simulink model "Const_VF_Openloop"  (R2023a)
settings: Solver=VariableStepAuto  StartTime=0.0  StopTime=10.0  MaxStep=.00001  RelTol=1e-3
values from neighbouring files (symbols this model uses):
  B = .005752    (= 0.005752)    [Parameters.m]
  J = .02    (= 0.02)    [Parameters.m]
  offset = Vph_p-(slope*Freq)    [Parameters.m]
  P = 4    [Parameters.m]
  slope = (Vph_p-VF_boost)/(Freq-1)    [Parameters.m]
  Te_rated = Prated/Wr_rated    (= 20.3536435794)    [Parameters.m]
  Vph_p = VLL_p/sqrt(3)    [Parameters.m]
  Wslip_rated = Ws_rated-Wr_rated    (= 5.23598775598)    [Parameters.m]
libraries: spsMosfetLib x12, spsAsynchronousMachineSIUnitsLib x2, spsDCVoltageSourceLib x2, slpidlib x2, spsTriangleGeneratorLib x2, SignalEditorBlockLib x1, sps_lib x1
settings Model: Creator=User  LastModifiedBy=User
settings SolverCC: ConsecutiveZCsStepRelTol=1000*128*eps  MaxConsecutiveZCs=2000
settings DebuggingCC: IgnoredZcDiagnostic=none

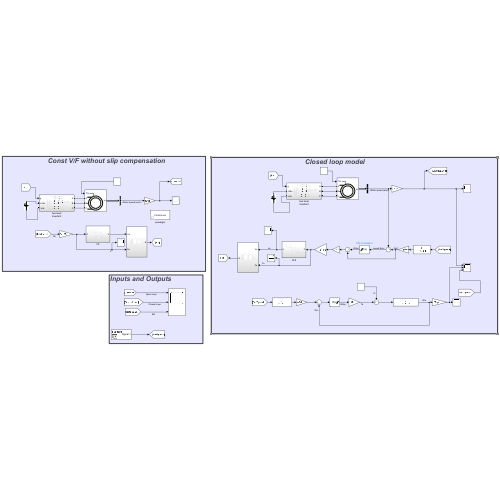
[thumbnail: Simulink's stored preview of the top-level diagram]
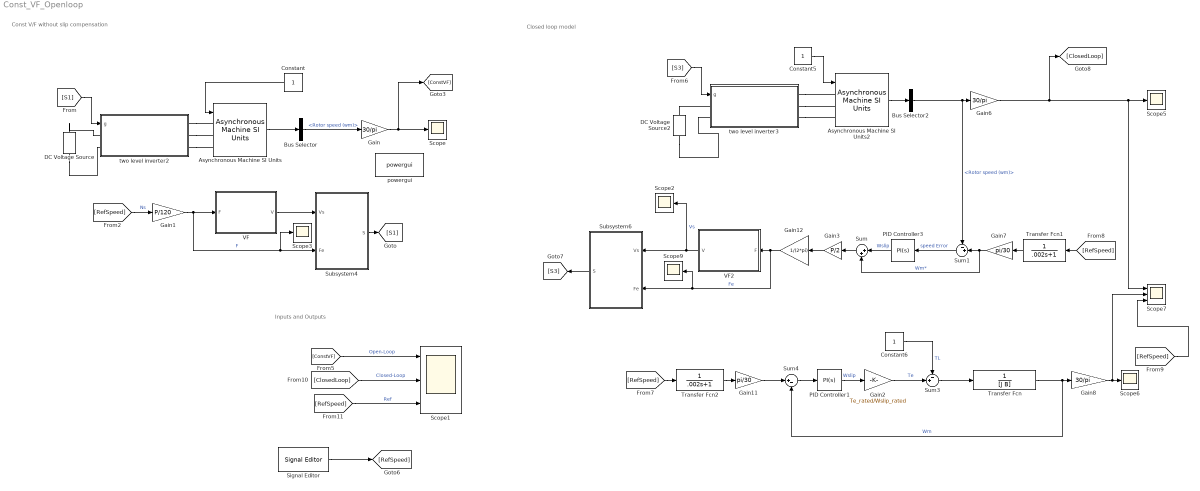
== system Const_VF_Openloop ==
  note: Inputs and Outputs
  note: Const V/F without slip compensation
  note: Closed loop model
  Asynchronous Machine SI Units : spsAsynchronousMachineSIUnitsLib/Asynchronous Machine SI Units  RotorType=Squirrel-cage  PresetModel="01:  5 HP   460 V 60Hz 1750 RPM"  MechanicalLoad=Torque Tm  ShowDetailedParameters=on  ReferenceFrame=Stationary  Units=SI  MeasurementBus=off  NominalParameters=[3730 460 60]  VoltageRatio=1  Stator=[1.115 0.005974]  Rotor=[1.083 0.005974]  Cage1=[0.4155 0.002066]  Cage2=[0.4168 0.0003495]  Lm=0.2037  Mechanical=[0.02 0.005752 2]  PolePairs=2  InitialConditions=[1 0 0 0 0 0 0 0]  SimulateSaturation=off  Saturation=[14.03593122, 27.81365428, 53.79336849, 72.68890987, 97.98006896, 148.6815601, 215.7428561, 302.9841135, 428.7778367 ; 230, 322, 414, 460, 506, 552, 598, 644, 690]  LoadFlowParameters=1492000  TsPowergui=0  TsBlock=-1  IterativeModel=Trapezoidal non iterative  IterativeDiscreteModel=Trapezoidal non iterative  Pmec=1.492e+006
  Asynchronous Machine SI Units2 : spsAsynchronousMachineSIUnitsLib/Asynchronous Machine SI Units  RotorType=Squirrel-cage  PresetModel="01:  5 HP   460 V 60Hz 1750 RPM"  MechanicalLoad=Torque Tm  ShowDetailedParameters=on  ReferenceFrame=Stationary  Units=SI  MeasurementBus=off  NominalParameters=[3730 460 60]  VoltageRatio=1  Stator=[1.115 0.005974]  Rotor=[1.083 0.005974]  Cage1=[0.4155 0.002066]  Cage2=[0.4168 0.0003495]  Lm=0.2037  Mechanical=[0.02 0.005752 2]  PolePairs=2  InitialConditions=[1 0 0 0 0 0 0 0]  SimulateSaturation=off  Saturation=[14.03593122, 27.81365428, 53.79336849, 72.68890987, 97.98006896, 148.6815601, 215.7428561, 302.9841135, 428.7778367 ; 230, 322, 414, 460, 506, 552, 598, 644, 690]  LoadFlowParameters=1492000  TsPowergui=0  TsBlock=-1  IterativeModel=Trapezoidal non iterative  IterativeDiscreteModel=Trapezoidal non iterative  Pmec=1.492e+006
  Bus Selector : BusSelector  OutputSignals=Mechanical.Rotor speed (wm)
  Bus Selector2 : BusSelector  OutputSignals=Mechanical.Rotor speed (wm)
  Constant : Constant
  Constant5 : Constant
  Constant6 : Constant
  DC Voltage Source : spsDCVoltageSourceLib/DC Voltage Source  Amplitude=Vph_p  Measurements=None
  DC Voltage Source2 : spsDCVoltageSourceLib/DC Voltage Source  Amplitude=Vph_p  Measurements=None
  Gain : Gain  Gain=30/pi
  Gain1 : Gain  Gain=P/120
  Gain11 : Gain  Gain=pi/30
  Gain12 : Gain  Gain=1/(2*pi)
  Gain2 : Gain  Gain=Te_rated/Wslip_rated
  Gain3 : Gain  Gain=P/2
  Gain6 : Gain  Gain=30/pi
  Gain7 : Gain  Gain=pi/30
  Gain8 : Gain  Gain=30/pi
  PID Controller1 : slpidlib/PID Controller  Controller=PI  Form=Parallel  TimeDomain=Continuous-time  UseExternalTs=off  SampleTime=-1  IntegratorMethod=Forward Euler  FilterMethod=Forward Euler  ControllerParametersSource=internal  P=2.61459800352204  I=169.186564549332  UseKiTs=off  D=0  N=100  UseFilter=on  TunerSelectOption=Transfer Function Based (PID Tuner App)  InitialConditionSource=internal  InitialConditionForIntegrator=0  InitialConditionForFilter=0  DifferentiatorICPrevScaledInput=0  ExternalReset=none  TrackingMode=off  Kt=1  LimitOutput=on  SatLimitsSource=internal  UpperSaturationLimit=Wslip_rated  LowerSaturationLimit=0  LinearizeAsGain=on  AntiWindupMode=clamping  Kb=1  LimitIntegrator=off  UpperIntegratorSaturationLimit=inf  LowerIntegratorSaturationLimit=-inf  POutMin=[]  POutMax=[]  IOutMin=[]  IOutMax=[]  DOutMin=[]  DOutMax=[]  NOutMin=[]  NOutMax=[]  SumOutMin=[]  SumOutMax=[]  SaturationOutMin=[]  SaturationOutMax=[]  PParamMin=[]  PParamMax=[]  IParamMin=[]  IParamMax=[]  DParamMin=[]  DParamMax=[]  NParamMin=[]  NParamMax=[]  KbParamMin=[]  KbParamMax=[]  KtParamMin=[]  KtParamMax=[]  KbOutMin=[]  KbOutMax=[]  KtOutMin=[]  KtOutMax=[]  IntegratorOutMin=[]  IntegratorOutMax=[]  FilterOutMin=[]  FilterOutMax=[]  SumI1OutMin=[]  SumI1OutMax=[]  SumI2OutMin=[]  SumI2OutMax=[]  SumI3OutMin=[]  SumI3OutMax=[]  SumI4OutMin=[]  SumI4OutMax=[]  SumDOutMin=[]  SumDOutMax=[]  DifferentiatorOutMin=[]  DifferentiatorOutMax=[]  FilterDiffOutCoefMin=[]  FilterDiffOutCoefMax=[]  ReciprocalOutMin=[]  ReciprocalOutMax=[]  SumDenOutMin=[]  SumDenOutMax=[]  SumNumOutMin=[]  SumNumOutMax=[]  DivideOutMin=[]  DivideOutMax=[]  UdiffTsProdOutMin=[]  UdiffTsProdOutMax=[]  NTsProdOutMin=[]  NTsProdOutMax=[]  UintegralTsProdOutMin=[]  UintegralTsProdOutMax=[]  UngainTsProdOutMin=[]  UngainTsProdOutMax=[]  ClampingZeroOutDataTypeStr=Inherit: Inherit via back propagation  ClampingZeroOutMin=[]  ClampingZeroOutMax=[]  FilterDenConstantOutDataTypeStr=Inherit: Inherit via back propagation  FilterDenConstantOutMin=[]  FilterDenConstantOutMax=[]  PCopyOutDataTypeStr=Inherit: Inherit via back propagation  PCopyOutMin=[]  PCopyOutMax=[]  NCopyOutDataTypeStr=Inherit: Inherit via back propagation  NCopyOutMin=[]  NCopyOutMax=[]  IntegratorContinuousStateAttributes=''  IntegratorStateMustResolveToSignalObject=off  IntegratorRTWStateStorageClass=Auto  FilterContinuousStateAttributes=''  FilterStateMustResolveToSignalObject=off  FilterRTWStateStorageClass=Auto  ParallelPVariant=InternalParameters  IdealPVariant=Disabled  IVariant=InternalParameters  DVariant=Disabled  IntegratorVariant=Continuous  SatVariant=Enabled  AWVariant=ContClampingParallel  PCopyVariant=Disabled  TRVariant=Disabled  FdbkBlocksVariant=Forward  IdealPFdbkVariant=Disabled  SatFdbkVariant=Disabled  DerivativeFilterVariant=Disabled  NVariant=Disabled  NCopyVariant=Disabled_SignalSpec  FilterICVariant=Disabled  IntegratorICVariant=InternalICs  ExternalResetVariant=Disabled  TRSumVariant=Passthrough  SumFdbkVariant=Disabled  SumVariant=Sum_PI  TsampFilterVariant=InternalTs  TsampNgainVariant=Passthrough  TsampIntegralVariant=Disabled_SignalSpec  ExternalSaturationOutDataTypeStr=Inherit: Same as second input
  PID Controller3 : slpidlib/PID Controller  Controller=PI  Form=Parallel  TimeDomain=Continuous-time  UseExternalTs=off  SampleTime=-1  IntegratorMethod=Forward Euler  FilterMethod=Forward Euler  ControllerParametersSource=internal  P=2.61459800352204  I=169.186564549332  UseKiTs=off  D=0  N=100  UseFilter=on  TunerSelectOption=Transfer Function Based (PID Tuner App)  InitialConditionSource=internal  InitialConditionForIntegrator=0  InitialConditionForFilter=0  DifferentiatorICPrevScaledInput=0  ExternalReset=none  TrackingMode=off  Kt=1  LimitOutput=on  SatLimitsSource=internal  UpperSaturationLimit=Wslip_rated  LowerSaturationLimit=0  LinearizeAsGain=on  AntiWindupMode=clamping  Kb=1  LimitIntegrator=off  UpperIntegratorSaturationLimit=inf  LowerIntegratorSaturationLimit=-inf  POutMin=[]  POutMax=[]  IOutMin=[]  IOutMax=[]  DOutMin=[]  DOutMax=[]  NOutMin=[]  NOutMax=[]  SumOutMin=[]  SumOutMax=[]  SaturationOutMin=[]  SaturationOutMax=[]  PParamMin=[]  PParamMax=[]  IParamMin=[]  IParamMax=[]  DParamMin=[]  DParamMax=[]  NParamMin=[]  NParamMax=[]  KbParamMin=[]  KbParamMax=[]  KtParamMin=[]  KtParamMax=[]  KbOutMin=[]  KbOutMax=[]  KtOutMin=[]  KtOutMax=[]  IntegratorOutMin=[]  IntegratorOutMax=[]  FilterOutMin=[]  FilterOutMax=[]  SumI1OutMin=[]  SumI1OutMax=[]  SumI2OutMin=[]  SumI2OutMax=[]  SumI3OutMin=[]  SumI3OutMax=[]  SumI4OutMin=[]  SumI4OutMax=[]  SumDOutMin=[]  SumDOutMax=[]  DifferentiatorOutMin=[]  DifferentiatorOutMax=[]  FilterDiffOutCoefMin=[]  FilterDiffOutCoefMax=[]  ReciprocalOutMin=[]  ReciprocalOutMax=[]  SumDenOutMin=[]  SumDenOutMax=[]  SumNumOutMin=[]  SumNumOutMax=[]  DivideOutMin=[]  DivideOutMax=[]  UdiffTsProdOutMin=[]  UdiffTsProdOutMax=[]  NTsProdOutMin=[]  NTsProdOutMax=[]  UintegralTsProdOutMin=[]  UintegralTsProdOutMax=[]  UngainTsProdOutMin=[]  UngainTsProdOutMax=[]  ClampingZeroOutDataTypeStr=Inherit: Inherit via back propagation  ClampingZeroOutMin=[]  ClampingZeroOutMax=[]  FilterDenConstantOutDataTypeStr=Inherit: Inherit via back propagation  FilterDenConstantOutMin=[]  FilterDenConstantOutMax=[]  PCopyOutDataTypeStr=Inherit: Inherit via back propagation  PCopyOutMin=[]  PCopyOutMax=[]  NCopyOutDataTypeStr=Inherit: Inherit via back propagation  NCopyOutMin=[]  NCopyOutMax=[]  IntegratorContinuousStateAttributes=''  IntegratorStateMustResolveToSignalObject=off  IntegratorRTWStateStorageClass=Auto  FilterContinuousStateAttributes=''  FilterStateMustResolveToSignalObject=off  FilterRTWStateStorageClass=Auto  ParallelPVariant=InternalParameters  IdealPVariant=Disabled  IVariant=InternalParameters  DVariant=Disabled  IntegratorVariant=Continuous  SatVariant=Enabled  AWVariant=ContClampingParallel  PCopyVariant=Disabled  TRVariant=Disabled  FdbkBlocksVariant=Forward  IdealPFdbkVariant=Disabled  SatFdbkVariant=Disabled  DerivativeFilterVariant=Disabled  NVariant=Disabled  NCopyVariant=Disabled_SignalSpec  FilterICVariant=Disabled  IntegratorICVariant=InternalICs  ExternalResetVariant=Disabled  TRSumVariant=Passthrough  SumFdbkVariant=Disabled  SumVariant=Sum_PI  TsampFilterVariant=InternalTs  TsampNgainVariant=Passthrough  TsampIntegralVariant=Disabled_SignalSpec  ExternalSaturationOutDataTypeStr=Inherit: Same as second input
  Scope{,2..3,5..6,9} (6 alike) : Scope
  Scope1 : Scope  NumInputPorts=3
  Scope7 : Scope  NumInputPorts=3
  Signal Editor : SignalEditorBlockLib/Signal Editor  FileName=speedRef.mat  ActiveScenario=Scenario  ActiveSignal=Signal 1  IsBus=off  OutputBusObjectStr=Bus: BusObject  SampleTime=0  Interpolate=off  ZeroCross=off  OutputAfterFinalValue=Setting to zero  Unit=inherit  PreserveSignalName=on  ApplySigPropsToAllScenarios=on
  Subsystem4 : Subsystem
  Subsystem6 : Subsystem
  Sum : Sum  Inputs=|++
  Sum1 : Sum  Inputs=-+|
  Sum3 : Sum  Inputs=-+|
  Sum4 : Sum  Inputs=|+-
  Transfer Fcn : TransferFcn  Denominator=[J B]
  Transfer Fcn1 : TransferFcn  Denominator=[.002 1]
  Transfer Fcn2 : TransferFcn  Denominator=[.002 1]
  VF : Subsystem
  VF2 : Subsystem
  powergui : sps_lib/powergui  Priority=1  SimulationMode=Continuous  SampleTime=50e-6  frequency=60  Iterations=50  frequencyindice=60  Pbase=100e6  ErrMax=1e-4  UnitsV=kV  UnitsW=MW  buscounter=0  FunctionMessages=off  echomessages=off  EnableUseOfTLC=off  CurrentSourceSwitches=off  DisableSnubberDevices=off  DisableRonSwitches=off  DisableVfSwitches=off  DisplayEquations=off  AutomaticDiscreteSolvers=off  SolverType=Tustin/Backward Euler (TBE)  Interpol=off  ExternalGateDelay=off  methode=off  Ts=100  x0status=blocks  SPID=on  SwTol=0  HookPort=off  NonlinearTolerance=1e-4  nMaxIteration=100  ContinueOnMaxIteration=off  RestoreLinks=warning  ResistiveCurrentMeasurement=off  Frange=[0:2:500]  Ylog=off  Xlog=on  ShowGrid=off  save=off  variable=ZData  structure=0  ZoomFFT=off  StartTime=0.0  cycles=1  DisplayStyle=1  fundamental=60  FreqAxis=off  MaxFrequency=1000  frequencyindicesteady=1  RmsSteady=1  display=off
  two level inverter2 : Subsystem
  two level inverter3 : Subsystem
  wires:
  Asynchronous Machine SI Units/1 -> Bus Selector/1
  Bus Selector/1 -> Gain/1  "<Rotor speed (wm)>"
  Gain/1 -> [ConstVF], Scope/1
  [RefSpeed] -> Gain1/1  "Ns"
  Gain1/1 -> Scope3/1, Subsystem4/2(Fe), VF/1(F)  "F"
  VF/1(V) -> Subsystem4/1(Vs)
  Constant/1 -> Asynchronous Machine SI Units/1
  Subsystem4/1(S) -> [S1]
  [S1] -> two level inverter2/1(g)
  [S3] -> two level inverter3/1(g)
  Constant5/1 -> Asynchronous Machine SI Units2/1
  Gain6/1 -> [ClosedLoop], Scope7/1, Scope5/1
  Bus Selector2/1 -> Sum1/1, Gain6/1  "<Rotor speed (wm)>"
  Asynchronous Machine SI Units2/1 -> Bus Selector2/1
  Signal Editor/1 -> [RefSpeed]
  Gain7/1 -> Sum/2, Sum1/2  "Wm*"
  Gain12/1 -> VF2/1(F), Subsystem6/2(Fe), Scope9/1  "Fe"
  Sum3/1 -> Transfer Fcn/1
  Constant6/1 -> Sum3/1  "TL"
  Transfer Fcn/1 -> Sum4/2, Gain8/1  "Wm"
  Sum4/1 -> PID Controller1/1
  PID Controller1/1 -> Gain2/1  "Wslip"
  Gain8/1 -> Scope7/2, Scope6/1
  Gain11/1 -> Sum4/1
  [RefSpeed] -> Transfer Fcn2/1
  [RefSpeed] -> Scope7/3
  VF2/1(V) -> Scope2/1, Subsystem6/1(Vs)  "Vs"
  Subsystem6/1(S) -> [S3]
  [ConstVF] -> Scope1/1  "Open-Loop"
  [ClosedLoop] -> Scope1/2  "Closed-Loop"
  [RefSpeed] -> Scope1/3  "Ref"
  [RefSpeed] -> Transfer Fcn1/1
  Gain2/1 -> Sum3/2  "Te"
  Sum1/1 -> PID Controller3/1  "speed Error"
  PID Controller3/1 -> Sum/1  "Wslip"
  Sum/1 -> Gain3/1
  Transfer Fcn1/1 -> Gain7/1
  Transfer Fcn2/1 -> Gain11/1
  Gain3/1 -> Gain12/1
  connections:
  two level inverter2/RConn1 -- Asynchronous Machine SI Units/LConn1
  two level inverter2/RConn2 -- Asynchronous Machine SI Units/LConn2
  DC Voltage Source/RConn1 -- two level inverter2/LConn1
  DC Voltage Source/LConn1 -- two level inverter2/LConn2
  two level inverter2/RConn3 -- Asynchronous Machine SI Units/LConn3
  two level inverter3/RConn3 -- Asynchronous Machine SI Units2/LConn3
  DC Voltage Source2/RConn1 -- two level inverter3/LConn1
  two level inverter3/RConn1 -- Asynchronous Machine SI Units2/LConn1
  two level inverter3/RConn2 -- Asynchronous Machine SI Units2/LConn2
  DC Voltage Source2/LConn1 -- two level inverter3/LConn2

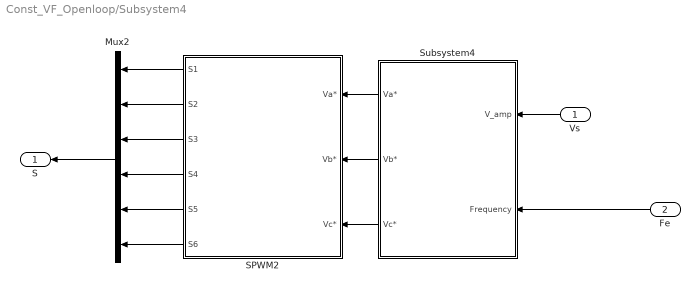
== system Const_VF_Openloop/Subsystem4 ==
  Vs : Inport
  Fe : Inport  Port=2
  Mux2 : Mux  Inputs=6
  SPWM2 : Subsystem
  Subsystem4 : Subsystem
  S : Outport
  wires:
  Mux2/1 -> S/1
  Fe/1 -> Subsystem4/2(Frequency)
  Vs/1 -> Subsystem4/1(V_amp)
  SPWM2/5(S5) -> Mux2/5
  Subsystem4/2(Vb*) -> SPWM2/2(Vb*)
  Subsystem4/1(Va*) -> SPWM2/1(Va*)
  SPWM2/6(S6) -> Mux2/6
  SPWM2/4(S4) -> Mux2/4
  SPWM2/1(S1) -> Mux2/1
  SPWM2/2(S2) -> Mux2/2
  SPWM2/3(S3) -> Mux2/3
  Subsystem4/3(Vc*) -> SPWM2/3(Vc*)

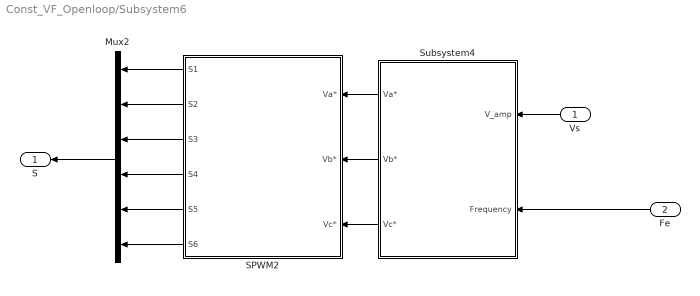
== system Const_VF_Openloop/Subsystem6 ==
  Vs : Inport
  Fe : Inport  Port=2
  Mux2 : Mux  Inputs=6
  SPWM2 : Subsystem
  Subsystem4 : Subsystem
  S : Outport
  wires:
  Subsystem4/3(Vc*) -> SPWM2/3(Vc*)
  SPWM2/3(S3) -> Mux2/3
  SPWM2/2(S2) -> Mux2/2
  SPWM2/1(S1) -> Mux2/1
  SPWM2/4(S4) -> Mux2/4
  SPWM2/6(S6) -> Mux2/6
  Subsystem4/1(Va*) -> SPWM2/1(Va*)
  Subsystem4/2(Vb*) -> SPWM2/2(Vb*)
  SPWM2/5(S5) -> Mux2/5
  Vs/1 -> Subsystem4/1(V_amp)
  Fe/1 -> Subsystem4/2(Frequency)
  Mux2/1 -> S/1

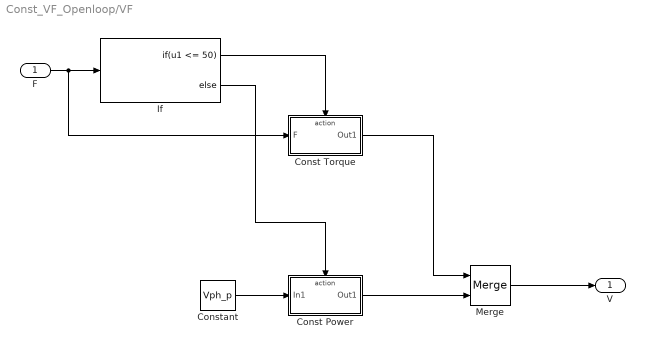
== system Const_VF_Openloop/VF ==
  F : Inport
  Const Power : Subsystem  TreatAsAtomicUnit=on
  Const Torque : Subsystem  TreatAsAtomicUnit=on
  Constant : Constant  Value=Vph_p
  If : If  IfExpression=u1 <= 50
  Merge : Merge
  V : Outport
  wires:
  F/1 -> Const Torque/1(F), If/1
  If/2 -> Const Power/Action
  Const Torque/1(Out1) -> Merge/1
  If/1 -> Const Torque/Action
  Merge/1 -> V/1
  Constant/1 -> Const Power/1(In1)
  Const Power/1(Out1) -> Merge/2

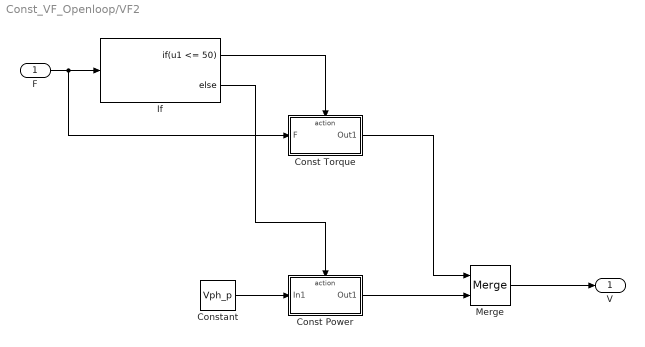
== system Const_VF_Openloop/VF2 ==
  F : Inport
  Const Power : Subsystem  TreatAsAtomicUnit=on
  Const Torque : Subsystem  TreatAsAtomicUnit=on
  Constant : Constant  Value=Vph_p
  If : If  IfExpression=u1 <= 50
  Merge : Merge
  V : Outport
  wires:
  Const Power/1(Out1) -> Merge/2
  Constant/1 -> Const Power/1(In1)
  Merge/1 -> V/1
  If/1 -> Const Torque/Action
  Const Torque/1(Out1) -> Merge/1
  If/2 -> Const Power/Action
  F/1 -> If/1, Const Torque/1(F)

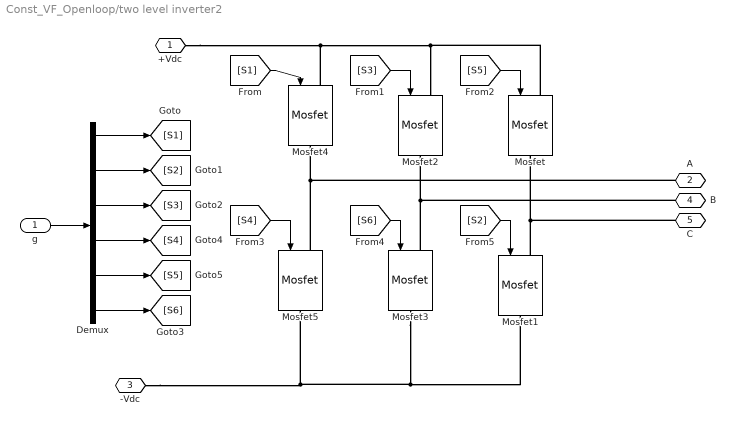
== system Const_VF_Openloop/two level inverter2 ==
  g : Inport
  Demux : Demux  Outputs=6
  Mosfet{,1..5} (6 alike) : spsMosfetLib/Mosfet  Ron=0.1  Lon=0  Rd=0.01  Vfd=0  IC=0  Rs=1e5  Cs=inf  Measurements=off
  +Vdc : PMIOPort  Side=Left
  A : PMIOPort  Port=2  Side=Right
  -Vdc : PMIOPort  Port=3  Side=Left
  B : PMIOPort  Port=4  Side=Right
  C : PMIOPort  Port=5  Side=Right
  wires:
  g/1 -> Demux/1
  Demux/1 -> [S1]
  Demux/2 -> [S2]
  Demux/3 -> [S3]
  Demux/4 -> [S4]
  Demux/5 -> [S5]
  Demux/6 -> [S6]
  [S1] -> Mosfet4/1
  [S3] -> Mosfet2/1
  [S5] -> Mosfet/1
  [S4] -> Mosfet5/1
  [S6] -> Mosfet3/1
  [S2] -> Mosfet1/1
  connections:
  Mosfet4/LConn1 -- +Vdc/RConn1 -- Mosfet/LConn1 -- Mosfet2/LConn1
  Mosfet3/RConn1 -- Mosfet1/RConn1 -- -Vdc/RConn1 -- Mosfet5/RConn1
  Mosfet1/LConn1 -- Mosfet/RConn1 -- C/RConn1
  Mosfet3/LConn1 -- B/RConn1 -- Mosfet2/RConn1
  A/RConn1 -- Mosfet5/LConn1 -- Mosfet4/RConn1

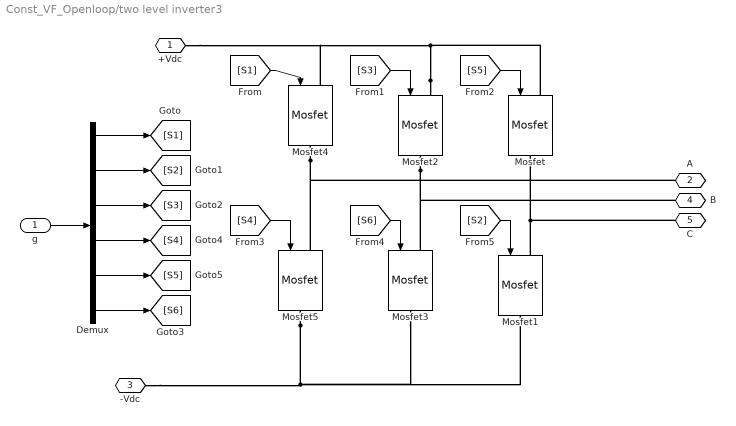
== system Const_VF_Openloop/two level inverter3 ==
  g : Inport
  Demux : Demux  Outputs=6
  Mosfet{,1..5} (6 alike) : spsMosfetLib/Mosfet  Ron=0.1  Lon=0  Rd=0.01  Vfd=0  IC=0  Rs=1e5  Cs=inf  Measurements=off
  +Vdc : PMIOPort  Side=Left
  A : PMIOPort  Port=2  Side=Right
  -Vdc : PMIOPort  Port=3  Side=Left
  B : PMIOPort  Port=4  Side=Right
  C : PMIOPort  Port=5  Side=Right
  wires:
  [S2] -> Mosfet1/1
  [S6] -> Mosfet3/1
  [S4] -> Mosfet5/1
  [S5] -> Mosfet/1
  [S3] -> Mosfet2/1
  [S1] -> Mosfet4/1
  Demux/6 -> [S6]
  Demux/5 -> [S5]
  Demux/4 -> [S4]
  Demux/3 -> [S3]
  Demux/2 -> [S2]
  Demux/1 -> [S1]
  g/1 -> Demux/1
  connections:
  Mosfet4/RConn1 -- Mosfet5/LConn1 -- A/RConn1
  Mosfet2/RConn1 -- B/RConn1 -- Mosfet3/LConn1
  C/RConn1 -- Mosfet/RConn1 -- Mosfet1/LConn1
  Mosfet5/RConn1 -- -Vdc/RConn1 -- Mosfet1/RConn1 -- Mosfet3/RConn1
  Mosfet2/LConn1 -- Mosfet/LConn1 -- +Vdc/RConn1 -- Mosfet4/LConn1

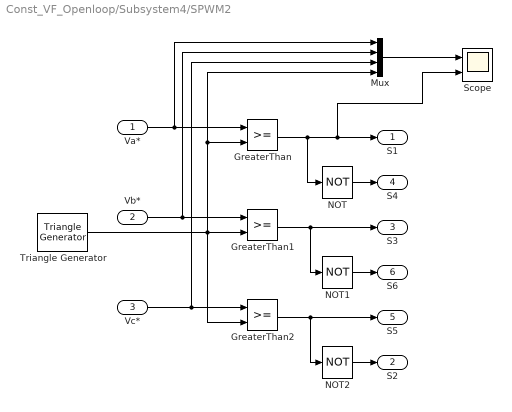
== system Const_VF_Openloop/Subsystem4/SPWM2 ==
  Va* : Inport
  Vb* : Inport  Port=2
  Vc* : Inport  Port=3
  GreaterThan : RelationalOperator  OutDataTypeStr=boolean  RndMeth=Simplest  InputSameDT=off
  GreaterThan1 : RelationalOperator  OutDataTypeStr=boolean  RndMeth=Simplest  InputSameDT=off
  GreaterThan2 : RelationalOperator  OutDataTypeStr=boolean  RndMeth=Simplest  InputSameDT=off
  Mux : Mux
  NOT : Logic  Operator=NOT  IconShape=distinctive  AllPortsSameDT=off  OutDataTypeStr=boolean
  NOT1 : Logic  Operator=NOT  IconShape=distinctive  AllPortsSameDT=off  OutDataTypeStr=boolean
  NOT2 : Logic  Operator=NOT  IconShape=distinctive  AllPortsSameDT=off  OutDataTypeStr=boolean
  Scope : Scope  NumInputPorts=2
  Triangle Generator : spsTriangleGeneratorLib/Triangle Generator  Freq=5e3  Phase=90  Ts=0
  S1 : Outport
  S2 : Outport  Port=2
  S3 : Outport  Port=3
  S4 : Outport  Port=4
  S5 : Outport  Port=5
  S6 : Outport  Port=6
  wires:
  Triangle Generator/1 -> GreaterThan2/2, GreaterThan1/2, Mux/4, GreaterThan/2
  Va*/1 -> Mux/1, GreaterThan/1
  Vb*/1 -> Mux/2, GreaterThan1/1
  Vc*/1 -> Mux/3, GreaterThan2/1
  GreaterThan/1 -> NOT/1, Scope/2, S1/1
  GreaterThan1/1 -> NOT1/1, S3/1
  GreaterThan2/1 -> NOT2/1, S5/1
  NOT/1 -> S4/1
  NOT1/1 -> S6/1
  NOT2/1 -> S2/1
  Mux/1 -> Scope/1

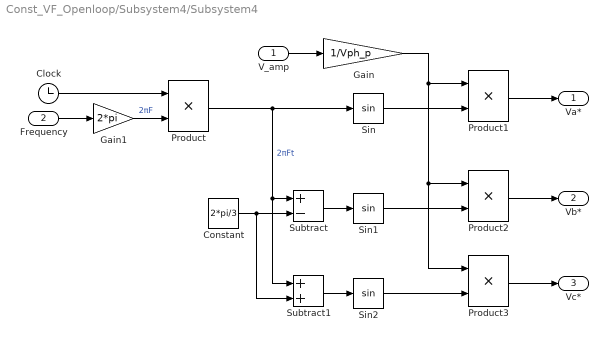
== system Const_VF_Openloop/Subsystem4/Subsystem4 ==
  V_amp : Inport
  Frequency : Inport  Port=2
  Clock : Clock
  Constant : Constant  Value=2*pi/3
  Gain : Gain  Gain=1/Vph_p
  Gain1 : Gain  Gain=2*pi
  Product{,1..3} (4 alike) : Product
  Sin : Trigonometry
  Sin1 : Trigonometry
  Sin2 : Trigonometry
  Subtract : Sum  Inputs=+-
  Subtract1 : Sum
  Va* : Outport
  Vb* : Outport  Port=2
  Vc* : Outport  Port=3
  wires:
  V_amp/1 -> Gain/1
  Frequency/1 -> Gain1/1
  Gain1/1 -> Product/2  "2πF"
  Clock/1 -> Product/1
  Product/1 -> Subtract1/1, Subtract/1, Sin/1  "2πFt"
  Subtract/1 -> Sin1/1
  Subtract1/1 -> Sin2/1
  Constant/1 -> Subtract1/2, Subtract/2
  Sin/1 -> Product1/2
  Gain/1 -> Product3/1, Product2/1, Product1/1
  Product1/1 -> Va*/1
  Sin1/1 -> Product2/2
  Sin2/1 -> Product3/2
  Product2/1 -> Vb*/1
  Product3/1 -> Vc*/1

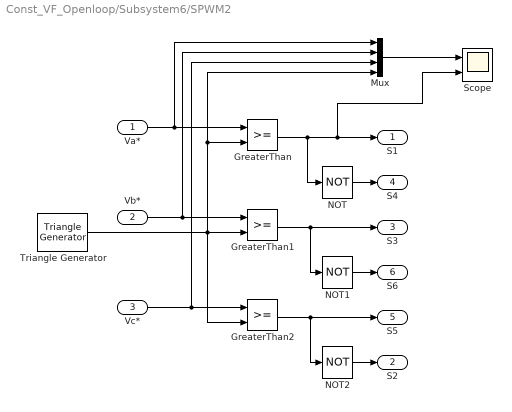
== system Const_VF_Openloop/Subsystem6/SPWM2 ==
  Va* : Inport
  Vb* : Inport  Port=2
  Vc* : Inport  Port=3
  GreaterThan : RelationalOperator  OutDataTypeStr=boolean  RndMeth=Simplest  InputSameDT=off
  GreaterThan1 : RelationalOperator  OutDataTypeStr=boolean  RndMeth=Simplest  InputSameDT=off
  GreaterThan2 : RelationalOperator  OutDataTypeStr=boolean  RndMeth=Simplest  InputSameDT=off
  Mux : Mux
  NOT : Logic  Operator=NOT  IconShape=distinctive  AllPortsSameDT=off  OutDataTypeStr=boolean
  NOT1 : Logic  Operator=NOT  IconShape=distinctive  AllPortsSameDT=off  OutDataTypeStr=boolean
  NOT2 : Logic  Operator=NOT  IconShape=distinctive  AllPortsSameDT=off  OutDataTypeStr=boolean
  Scope : Scope  NumInputPorts=2
  Triangle Generator : spsTriangleGeneratorLib/Triangle Generator  Freq=5e3  Phase=90  Ts=0
  S1 : Outport
  S2 : Outport  Port=2
  S3 : Outport  Port=3
  S4 : Outport  Port=4
  S5 : Outport  Port=5
  S6 : Outport  Port=6
  wires:
  Mux/1 -> Scope/1
  NOT2/1 -> S2/1
  NOT1/1 -> S6/1
  NOT/1 -> S4/1
  GreaterThan2/1 -> S5/1, NOT2/1
  GreaterThan1/1 -> S3/1, NOT1/1
  GreaterThan/1 -> S1/1, Scope/2, NOT/1
  Vc*/1 -> GreaterThan2/1, Mux/3
  Vb*/1 -> GreaterThan1/1, Mux/2
  Va*/1 -> GreaterThan/1, Mux/1
  Triangle Generator/1 -> GreaterThan/2, Mux/4, GreaterThan1/2, GreaterThan2/2

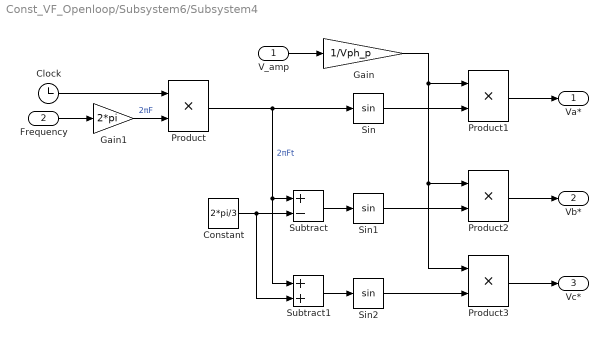
== system Const_VF_Openloop/Subsystem6/Subsystem4 ==
  V_amp : Inport
  Frequency : Inport  Port=2
  Clock : Clock
  Constant : Constant  Value=2*pi/3
  Gain : Gain  Gain=1/Vph_p
  Gain1 : Gain  Gain=2*pi
  Product{,1..3} (4 alike) : Product
  Sin : Trigonometry
  Sin1 : Trigonometry
  Sin2 : Trigonometry
  Subtract : Sum  Inputs=+-
  Subtract1 : Sum
  Va* : Outport
  Vb* : Outport  Port=2
  Vc* : Outport  Port=3
  wires:
  Product3/1 -> Vc*/1
  Product2/1 -> Vb*/1
  Sin2/1 -> Product3/2
  Sin1/1 -> Product2/2
  Product1/1 -> Va*/1
  Gain/1 -> Product1/1, Product2/1, Product3/1
  Sin/1 -> Product1/2
  Constant/1 -> Subtract/2, Subtract1/2
  Subtract1/1 -> Sin2/1
  Subtract/1 -> Sin1/1
  Product/1 -> Sin/1, Subtract/1, Subtract1/1  "2πFt"
  Clock/1 -> Product/1
  Gain1/1 -> Product/2  "2πF"
  Frequency/1 -> Gain1/1
  V_amp/1 -> Gain/1

== system Const_VF_Openloop/VF/Const Power ==
  In1 : Inport
  Action Port : ActionPort  ActionPortLabel=else
  Out1 : Outport
  wires:
  In1/1 -> Out1/1

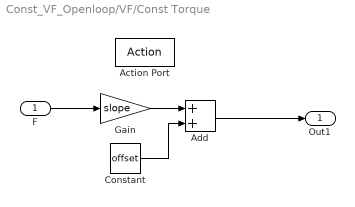
== system Const_VF_Openloop/VF/Const Torque ==
  F : Inport
  Action Port : ActionPort  ActionPortLabel=if(u1 <= 50)
  Add : Sum
  Constant : Constant  Value=offset
  Gain : Gain  Gain=slope
  Out1 : Outport
  wires:
  F/1 -> Gain/1
  Gain/1 -> Add/1
  Add/1 -> Out1/1
  Constant/1 -> Add/2

== system Const_VF_Openloop/VF2/Const Power ==
  In1 : Inport
  Action Port : ActionPort  ActionPortLabel=else
  Out1 : Outport
  wires:
  In1/1 -> Out1/1

== system Const_VF_Openloop/VF2/Const Torque ==
  F : Inport
  Action Port : ActionPort  ActionPortLabel=if(u1 <= 50)
  Add : Sum
  Constant : Constant  Value=offset
  Gain : Gain  Gain=slope
  Out1 : Outport
  wires:
  Constant/1 -> Add/2
  Add/1 -> Out1/1
  Gain/1 -> Add/1
  F/1 -> Gain/1
